simulink model "BEV_system_model"  (R2023a)
settings: Solver=daessc  StartTime=0  StopTime=2474  MaxStep=0.1  RelTol=1e-3  AbsTol=1e-3  EnableMultiTasking=on
PreLoadFcn:
  | defineBus_HighVoltage
  | defineBus_Rotational
PostLoadFcn:
  | BEV_setup
undefined symbols (not defined in the file): Ion, Lithium, Minus, Plus
libraries: spsMosfetLib x4, slpidlib x4, spsCurrentMeasurementLib x2, spsSeriesRLCBranchLib x2, spsVoltageMeasurementLib x2, nesl_utility x2, spsBatteryLib x1, fl_lib x1, simulink x1, spsSupercapacitorLib x1, spspowerguiLib x1
Description:
  | Battery Electric Vehicle drive cycle simulation
settings Model: Creator=MathWorks  LastModifiedBy=antaeug
settings SolverCC: AutoScaleAbsTol=off  AlgebraicLoopSolver=TrustRegion  MinimalZcImpactIntegration=on
settings DataIOCC: MaxDataPoints=15000  SaveFormat=Array  DSMLogging=off
settings OptimizationCC: ReuseModelBlockBuffer=off  ExpressionDepthLimit=2147483647  LifeSpan=inf
settings DebuggingCC: UnderspecifiedInitializationDetection=Classic  MergeDetectMultiDrivingBlocksExec=none  FcnCallInpInsideContextMsg=warning  UnconnectedInputMsg=warning  UnconnectedOutputMsg=warning  UnconnectedLineMsg=warning  StateNameClashWarn=warning  SFUnexpectedBacktrackingDiag=warning  SFNoUnconditionalDefaultTransitionDiag=warning  SFExecutionAtInitializationDiag=none  UnitsInconsistencyMsg=none  ArithmeticOperatorsInVariantConditions=warning
settings HardwareCC: ProdBitPerPointer=32  ProdBitPerSizeT=32  ProdBitPerPtrDiffT=32  ProdLargestAtomicFloat=None  ProdIntDivRoundTo=Undefined  ProdEndianess=Unspecified  ProdWordSize=32  ProdHWDeviceType=32-bit Generic
settings ModelReferenceCC: EnableRefExpFcnMdlSchedulingChecks=on  PropagateSignalLabelsOutOfModel=off
settings SFSimCC: SimUseLocalCustomCode=off  CustomCodeUndefinedFunction=UseInterfaceOnly
settings RTWCC: RTWUseLocalCustomCode=off  DLArmComputeVersion=19.05
settings CodeAppCC: StateflowObjectComments=on
settings GRTTargetCC: TargetLangStandard=C89/C90 (ANSI)  CombineOutputUpdateFcns=off  GRTInterface=on
settings ConfigComp: CovScope=Subsystem  CovPath=Driver & Environment/Torque Limiter  CovMetricSettings=dcmw  CovSaveCumulativeToWorkspaceVar=on  CovSaveSingleToWorkspaceVar=on  CovExternalEMLEnable=off
settings SimscapeCC: SimscapeNominalValues="[{\"value\":\"20\",\"unit\":\"A\"},{\"value\":\"1\",\"unit\":\"bar\"},{\"value\":\"1\",\"unit\":\"cm^2\"},{\"value\":\"1\",\"unit\":\"cm^3/s\"},{\"value\":\"1\",\"unit\":\"kJ/kg\"},{\"value\":\"1\",\"unit\":\"kW\"},{\"value\":\"1\",\"unit\":\"l\"},{\"value\":\"1\",\"unit\":\"N\"},{\"value\":\"40\",\"unit\":\"N*m\"},{\"value\":\"350\",\"unit\":\"V\"}]"  SimscapeLogType=all  SimscapeLogSimulationStatistics=on  SimscapeLogName=logoutssc  SimscapeLogLimitData=off  SimscapeLogDataHistory=10000

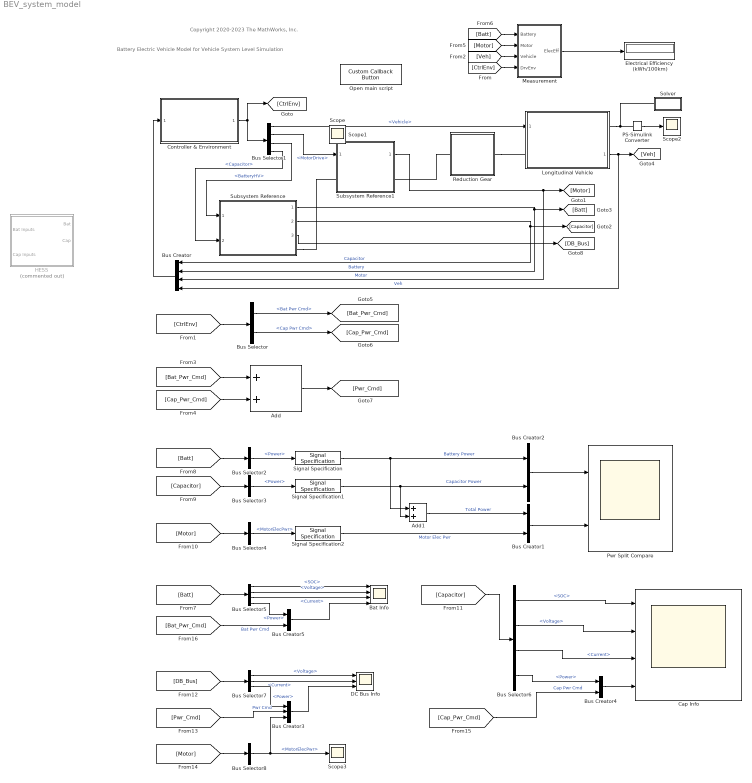
== system BEV_system_model ==
  note: Battery Electric Vehicle Model for Vehicle System Level Simulation
  note: Copyright 2020-2023 The MathWorks, Inc.
  Add : Sum
  Add1 : Sum
  Bat Info : Scope  NumInputPorts=4
  Bus Creator : BusCreator  Inputs=4
  Bus Creator{1..2,4..5} (4 alike) : BusCreator  Inputs=2
  Bus Creator3 : BusCreator  Inputs=3
  Bus Selector : BusSelector  OutputSignals=BatteryHV.Bat Pwr Cmd,Capacitor.Cap Pwr Cmd
  Bus Selector1 : BusSelector  OutputSignals=Vehicle,MotorDrive,BatteryHV,Capacitor
  Bus Selector2 : BusSelector  OutputSignals=Power
  Bus Selector3 : BusSelector  OutputSignals=Power
  Bus Selector4 : BusSelector  OutputSignals=MotorElecPwr
  Bus Selector5 : BusSelector  OutputSignals=SOC,Voltage,Current,Power
  Bus Selector6 : BusSelector  OutputSignals=SOC,Voltage,Current,Power
  Bus Selector7 : BusSelector  OutputSignals=Voltage,Current,Power
  Bus Selector8 : BusSelector  OutputSignals=MotorElecPwr
  Cap Info : Scope  NumInputPorts=4
  Controller & Environment : Subsystem  ReferencedSubsystem=CtrlEnv_refsub_Basic
      settings: OpenFcn=|
      | % Look under mask:
      | open_system(gcb, "force")
  DC Bus Info : Scope  NumInputPorts=3
  Electrical Efficiency (kWh/100km) : Display
  HESS : Subsystem  Commented=on
  Longitudinal Vehicle : Subsystem  ReferencedSubsystem=Vehicle1D_refsub_Basic
      settings: PortSchema="{\"entries\":[{\"content\":{\"sides\":[{\"content\":{\"connectorIds\":[\"In1\",\"LConn1\"]},\"type\":\"ConnectorPlacement.EquallySpacedRectSide\",\"uuid\":\"1278221b-4210-4fc4-9018-d7f4555b8d65\"},{\"content\":{\"connectorIds\":[\"RConn1\",\"Out1\"],\"side\":\"RIGHT\"},\"type\":\"ConnectorPlacement.EquallySpacedRectSide\",\"uuid\":\"ae02a7d1-22cf-4294-9907-02c3616e735c\"},{\"content\":{\"side\":\"TOP\"},\"type\":\"ConnectorPlacement.EquallySpacedRectSide\",\"uuid\":\"498bee53-b001-4331-968a-8dad39da1579\"}]},\"type\":\"ConnectorPlacement.EquallySpacedConnector\",\"uuid\":\"c28a1585-5582-45c2-8974-ffffcb6069ab\"}],\"packageUris\":[\"http://schema.mathworks.com/mf0/Connector/R2020b\"],\"version\":\"1.0\"}"
      settings: OpenFcn=|
      | % Look under mask:
      | open_system(gcb, "force")
  Measurement : Subsystem
  Open main script : CustomCallbackButton  Configuration="{\"components\":[{\"name\":\"BackgroundImageComponent\",\"settings\":{\"image\":{\"size\":[0,0],\"src\":\"default\",\"srcOrientation\":\"Right\"},\"position\":[0,0,1,1]}},{\"name\":\"ButtonStateComponent\",\"settings\":{\"buttonType\":\"momentary\",\"clickFcn\":\"edit(\\\"BEV_main_script\\\")\\n\",\"onValue\":1,\"position\":[0,0,1,1],\"pressDelay\":\"500\",\"pressFcn\":\"\",\"repeatInterval\":\"0\",\"states\":[{\"horizontalAlignment\":\"center\",\"image\":{\"position\":[0,0,1,1],\"src\":\"default\",\"srcOrientation\":\"Right\"},\"label\":{\"color\":[0.01176470588,0.01176470588,0.01176470588,1],\"icon\":{\"size\":[0,0],\"src\":\"default\",\"srcOrientation\":\"Right\"},\"iconPlacement\":\"left\",\"text\":{\"content\":\"Main script\"}},\"labelOffset\":[0,0],\"verticalAlignment\":\"middle\"},{\"horizontalAlignment\":\"center\",\"image\":{\"position\":[0,0,1,1],\"src\":\"default\",\"srcOrientation\":\"Right\"},\"label\":{\"color\":[0.01176470588,0.01176470588,0.01176470588,1],\"icon\":{\"size\":[0,0],\"src\":\"default\",\"srcOrientation\":\"Right\"},\"iconPlacement\":\"left\",\"text\":{\"content\":\"Main script\"}},\"labelOffset\":[0,0],\"verticalAlignment\":\"middle\"},{\"horizontalAlignment\":\"center\",\"image\":{\"position\":[0,0,1,1],\"src\":\"default\",\"srcOrientation\":\"Right\"},\"label\":{\"color\":[0.01176470588,0.01176470588,0.01176470588,1],\"icon\":{\"size\":[0,0],\"src\":\"default\",\"srcOrientation\":\"Right\"},\"iconPlacement\":\"left\",\"text\":{\"content\":\"Main script\"}},\"labelOffset\":[0,0],\"verticalAlignment\":\"middle\"},{\"horizontalAlignment\":\"center\",\"image\":{\"position\":[0,0,1,1],\"src\":\"default\",\"srcOrientation\":\"Right\"},\"label\":{\"color\":[0.01176470588,0.01176470588,0.01176470588,1],\"icon\":{\"size\":[0,0],\"src\":\"default\",\"srcOrientation\":\"Right\"},\"iconPlacement\":\"left\",\"text\":{\"content\":\"Main script\"}},\"labelOffset\":[0,0],\"verticalAlignment\":\"middle\"}]}},{\"name\":\"ForegroundImageComponent\",\"settings\":{\"image\":{\"size\":[0,0],\"src\":\"default\",\"srcOrientation\":\"Right\"},\"isForeground\":1,\"position\":[0,0,1,1]}}],\"settings\":{\"BindingType\":\"standalone\",\"backgroundColor\":[244,244,244,1],\"backgroundOffset\":0.2,\"backgroundOpacity\":1,\"fixedAspectRatio\":\"off\",\"foregroundColor\":[0.01176470588,0.01176470588,0.01176470588,1],\"migratedFromLegacy\":true,\"useBackgroundColor\":true,\"variant\":\"callback\",\"version\":\"R2023a\"},\"type\":\"Button\"}"  CustomBackgroundColor="{\"color\":[0.9568627451,0.9568627451,0.9568627451],\"show\":true}"
  PS-Simulink Converter : nesl_utility/PS-Simulink Converter  PhysicalDomain=network_engine_domain  SubClassName=ps_output  LeftPortType=input  RightPortType=output  PseudoPeriodic=off  Frequencies=[]  VectorFormat=inherit  Unit=m/s  AffineConversion=off
  Pwr Split Compare : Scope  NumInputPorts=2
  Reduction Gear : Subsystem  ReferencedSubsystem=Reducer_refsub_Basic
      settings: OpenFcn=|
      | % Look under mask:
      | open_system(gcb, "force")
  Scope{,1..3} (4 alike) : Scope
  Signal Specification : SignalSpecification  Unit=W
  Signal Specification1 : SignalSpecification  Unit=W
  Signal Specification2 : SignalSpecification  Unit=W
  Solver : Subsystem
  Subsystem Reference : Subsystem  ReferencedSubsystem=BatteryHV_refsub_System
  Subsystem Reference1 : Subsystem  ReferencedSubsystem=MotorDriveUnit_refsub_System
  wires:
  [Veh] -> Measurement/3(Vehicle)
  [Motor] -> Measurement/2(Motor)
  [Batt] -> Measurement/1(Battery)
  Subsystem Reference/1 -> Bus Creator/2, [Batt]  "Battery"
  Longitudinal Vehicle/1 -> [Veh], Bus Creator/4  "Veh"
  [CtrlEnv] -> Measurement/4(DrvEnv)
  Bus Selector1/2 -> Subsystem Reference1/1  "<MotorDrive>"
  Subsystem Reference1/1 -> Bus Creator/3, [Motor]  "Motor"
  Bus Creator/1 -> Controller & Environment/1
  Bus Selector1/3 -> Subsystem Reference/1  "<BatteryHV>"
  Bus Selector1/1 -> Longitudinal Vehicle/1  "<Vehicle>"
  Measurement/1(ElecEff) -> Electrical Efficiency (kWh/100km)/1
  Controller & Environment/1 -> Bus Selector1/1, [CtrlEnv]
  PS-Simulink Converter/1 -> Scope2/1
  Subsystem Reference/2 -> Bus Creator/1, [Capacitor]  "Capacitor"
  Bus Selector1/4 -> Subsystem Reference/2  "<Capacitor>"
  [CtrlEnv] -> Bus Selector/1
  Bus Selector/1 -> [Bat_Pwr_Cmd]  "<Bat Pwr Cmd>"
  Bus Selector/2 -> [Cap_Pwr_Cmd]  "<Cap Pwr Cmd>"
  [Bat_Pwr_Cmd] -> Add/1
  [Cap_Pwr_Cmd] -> Add/2
  Add/1 -> [Pwr_Cmd]
  [Batt] -> Bus Selector2/1
  [Capacitor] -> Bus Selector3/1
  Bus Selector2/1 -> Signal Specification/1  "<Power>"
  Bus Selector3/1 -> Signal Specification1/1  "<Power>"
  Add1/1 -> Bus Creator1/1  "Total Power"
  Bus Creator2/1 -> Pwr Split Compare/1
  Signal Specification/1 -> Add1/1, Bus Creator2/1  "Battery Power"
  Signal Specification1/1 -> Bus Creator2/2, Add1/2  "Capacitor Power"
  Bus Creator1/1 -> Pwr Split Compare/2
  [Motor] -> Bus Selector4/1
  Bus Selector4/1 -> Signal Specification2/1  "<MotorElecPwr>"
  Signal Specification2/1 -> Bus Creator1/2  "Motor Elec Pwr"
  [Batt] -> Bus Selector5/1
  Bus Selector5/2 -> Bat Info/2  "<Voltage>"
  Bus Selector5/1 -> Bat Info/1  "<SOC>"
  Bus Selector5/3 -> Bat Info/3  "<Current>"
  [Capacitor] -> Bus Selector6/1
  Subsystem Reference/3 -> [DB_Bus]
  [DB_Bus] -> Bus Selector7/1
  Bus Selector7/1 -> DC Bus Info/1  "<Voltage>"
  Bus Selector7/2 -> DC Bus Info/2  "<Current>"
  Bus Creator3/1 -> DC Bus Info/3
  Bus Selector7/3 -> Bus Creator3/1  "<Power>"
  [Pwr_Cmd] -> Bus Creator3/2  "Pwr Cmd"
  [Motor] -> Bus Selector8/1
  Bus Selector8/1 -> Bus Creator3/3, Scope3/1  "<MotorElecPwr>"
  Bus Selector6/1 -> Cap Info/1  "<SOC>"
  Bus Selector6/2 -> Cap Info/2  "<Voltage>"
  Bus Selector6/3 -> Cap Info/3  "<Current>"
  Bus Selector6/4 -> Bus Creator4/1  "<Power>"
  [Cap_Pwr_Cmd] -> Bus Creator4/2  "Cap Pwr Cmd"
  Bus Creator4/1 -> Cap Info/4
  Bus Selector5/4 -> Bus Creator5/1  "<Power>"
  Bus Creator5/1 -> Bat Info/4
  [Bat_Pwr_Cmd] -> Bus Creator5/2  "Bat Pwr Cmd"
  connections:
  Reduction Gear/RConn1 -- Longitudinal Vehicle/LConn1
  Reduction Gear/LConn1 -- Subsystem Reference1/RConn1
  Longitudinal Vehicle/RConn1 -- Solver/LConn1 -- PS-Simulink Converter/LConn1
  Subsystem Reference/RConn1 -- Subsystem Reference1/LConn1

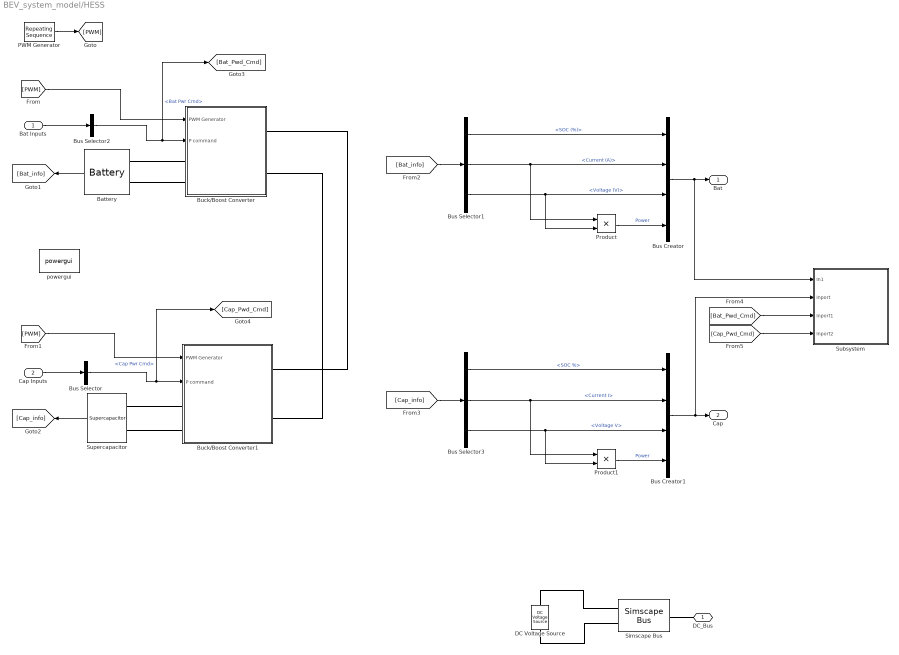
== system BEV_system_model/HESS ==
  Bat Inputs : Inport
  Cap Inputs : Inport  Port=2
  Battery : spsBatteryLib/Battery  BatType=Lithium-Ion  ShowTempParam=off  ThermalPreset=no  ShowAgeParam=off  NomV=300  NomQ=93.6  SOC=100  Batt_Tr=30  PresetModel=on  MaxQ=93.6  MinV=225  FullV=349.1961  Dis_rate=40.6957  R=0.032051  Normal_OP=84.647  expZone="[324.1158      4.598609]"  current=[6.5 13 32.5]  Units=Time  Tci=20  NomT=20  T2=-30  MaxQ2=4.8  FullV2=7.1  Normal_OP2=5.655  expZone2="[6.58           1]"  Rca=0.6  ti=2000  Dp=0  Neq0=0  Tsim=1e6  Ta1=25  Qeol=5.4*0.9  Reol=0.013333*1.2  Char_age=[2.3478, 3]  Dis_age=[2.3478, 10]  N1=1500  N2=10500  N3=1000  N4=1400  Ta2=45  N5=950
  Buck/Boost Converter : Subsystem
  Buck/Boost Converter1 : Subsystem
  Bus Creator : BusCreator  Inputs=4
  Bus Creator1 : BusCreator  Inputs=4
  Bus Selector : BusSelector  OutputSignals=Cap Pwr Cmd
  Bus Selector1 : BusSelector  OutputSignals=SOC (%),Current (A),Voltage (V)
  Bus Selector2 : BusSelector  OutputSignals=Bat Pwr Cmd
  Bus Selector3 : BusSelector  OutputSignals=SOC %,Current I,Voltage V
  DC Voltage Source : fl_lib/Electrical/Electrical Sources/DC Voltage Source  v0=300 V
  PWM Generator : simulink/Sources/Repeating Sequence  rep_seq_t="[0 1/4*0.0001  2/4*0.0001  3/4*0.0001  0.0001]"  rep_seq_y=[0 1 0 -1 0]
  Product : Product
  Product1 : Product
  Simscape Bus : SimscapeBus  HierarchyStrings=Plus;Minus  ConnectionType=Bus: Bus_HighVoltage
  Subsystem : Subsystem
  Supercapacitor : spsSupercapacitorLib/Supercapacitor  C=1500  Rdc=0.00047  Voltage=2.7  Ns=222  Np=1  Vinit=2.7  Temp=25  PresetModel=off  EstParam=off  Nc=1  r=1e-9  epsilon=6.0208e-10  Ich=10  Vstern="[0.161  2.7  7.8]"  Self_dis=on  Ioc=10  Vself="[48  47.8  47.06  44.65]"  demandeplot=off  I="[10  20 100  500]"  Units=sec  Vmax=0  If=0  deltaV=0  alpha=0  sec=0
      settings: LibrarySourceBlock=sps_lib/Sources/Supercapacitor
  powergui : spspowerguiLib/powergui  Priority=1  SimulationMode=Discrete  SampleTime=25e-6  frequency=60  Iterations=50  frequencyindice=0  Pbase=100e6  ErrMax=1e-4  UnitsV=kV  UnitsW=MW  buscounter=0  FunctionMessages=off  echomessages=off  EnableUseOfTLC=off  CurrentSourceSwitches=off  DisableSnubberDevices=off  DisableRonSwitches=off  DisableVfSwitches=off  DisplayEquations=off  AutomaticDiscreteSolvers=off  SolverType=Tustin/Backward Euler (TBE)  Interpol=off  ExternalGateDelay=off  methode=off  Ts=0  x0status=blocks  SPID=off  SwTol=0  HookPort=off  NonlinearTolerance=1e-4  nMaxIteration=100  ContinueOnMaxIteration=off  RestoreLinks=warning  ResistiveCurrentMeasurement=off  Frange=[0:1:1000]  Ylog=on  Xlog=on  ShowGrid=on  save=on  variable=ZDa  structure=donnee  ZoomFFT=off  StartTime=0.0  cycles=1  DisplayStyle=1  fundamental=60  FreqAxis=off  MaxFrequency=1000  frequencyindicesteady=10  RmsSteady=1  display=off
  DC_Bus : PMIOPort  Side=Right
  Bat : Outport
  Cap : Outport  Port=2
  wires:
  Bat Inputs/1 -> Bus Selector2/1
  Cap Inputs/1 -> Bus Selector/1
  PWM Generator/1 -> [PWM]
  Battery/1 -> [Bat_info]
  Supercapacitor/1 -> [Cap_info]
  Bus Selector2/1 -> [Bat_Pwd_Cmd], Buck/Boost Converter/2(P command)  "<Bat Pwr Cmd>"
  [PWM] -> Buck/Boost Converter/1(PWM Generator)
  Bus Selector/1 -> [Cap_Pwd_Cmd], Buck/Boost Converter1/2(P command)  "<Cap Pwr Cmd>"
  [PWM] -> Buck/Boost Converter1/1(PWM Generator)
  [Bat_info] -> Bus Selector1/1
  Bus Creator/1 -> Subsystem/1(In1), Bat/1
  Bus Selector1/1 -> Bus Creator/1  "<SOC (%)>"
  Bus Selector1/2 -> Product/1, Bus Creator/2  "<Current (A)>"
  Bus Selector1/3 -> Product/2, Bus Creator/3  "<Voltage (V)>"
  [Cap_info] -> Bus Selector3/1
  Bus Selector3/3 -> Product1/2, Bus Creator1/3  "<Voltage V>"
  Bus Selector3/2 -> Product1/1, Bus Creator1/2  "<Current I>"
  Product1/1 -> Bus Creator1/4  "Power"
  Bus Selector3/1 -> Bus Creator1/1  "<SOC %>"
  Bus Creator1/1 -> Subsystem/2(Inport), Cap/1
  [Bat_Pwd_Cmd] -> Subsystem/3(Inport1)
  [Cap_Pwd_Cmd] -> Subsystem/4(Inport2)
  Product/1 -> Bus Creator/4  "Power"
  connections:
  DC_Bus/RConn1 -- Simscape Bus/RConn1
  Buck/Boost Converter/LConn1 -- Battery/LConn1
  Buck/Boost Converter/LConn2 -- Battery/LConn2
  Buck/Boost Converter1/LConn1 -- Supercapacitor/LConn1
  Supercapacitor/LConn2 -- Buck/Boost Converter1/LConn2
  Buck/Boost Converter/RConn1 -- Buck/Boost Converter1/RConn1
  Buck/Boost Converter/RConn2 -- Buck/Boost Converter1/RConn2
  DC Voltage Source/LConn1 -- Simscape Bus/LConn1
  DC Voltage Source/RConn1 -- Simscape Bus/LConn2

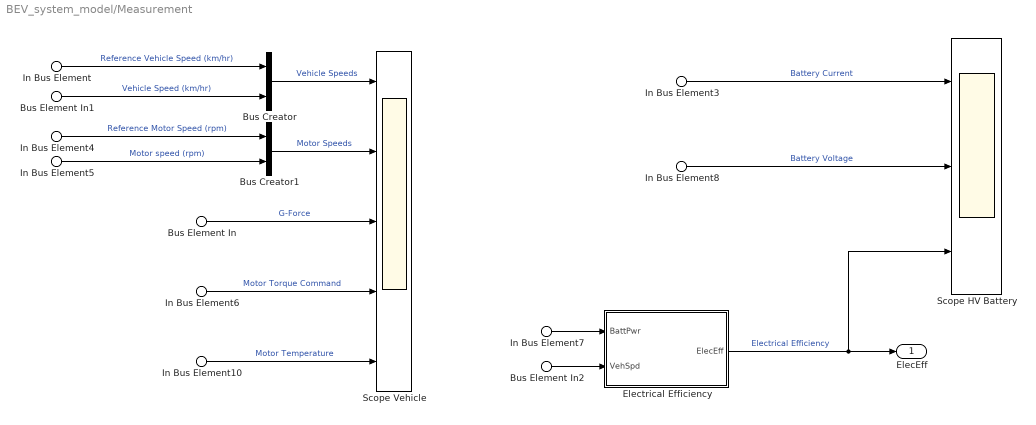
== system BEV_system_model/Measurement ==
  In Bus Element3 : Inport  PortName=Battery  Element=Current
  In Bus Element7 : Inport  PortName=Battery  Element=Power
  In Bus Element8 : Inport  PortName=Battery  Element=Voltage
  In Bus Element6 : Inport  Port=2  PortName=Motor  Element=TrqCmd
  In Bus Element5 : Inport  Port=2  PortName=Motor  Element=MotorSpd
  In Bus Element10 : Inport  Port=2  PortName=Motor  Element=MotorTemp
  Bus Element In : Inport  Port=3  PortName=Vehicle  Element=G
  Bus Element In2 : Inport  Port=3  PortName=Vehicle  Element=VehSpdKph
  Bus Element In1 : Inport  Port=3  PortName=Vehicle  Element=VehSpdKph
  In Bus Element : Inport  Port=4  PortName=DrvEnv  Element=Info.VehSpdRef
  In Bus Element4 : Inport  Port=4  PortName=DrvEnv  Element=Info.MotorSpdRef
  Bus Creator : BusCreator  Inputs=2
  Bus Creator1 : BusCreator  Inputs=2
  Electrical Efficiency : Subsystem
  Scope HV Battery : Scope  NumInputPorts=3
  Scope Vehicle : Scope  NumInputPorts=5
  ElecEff : Outport
  wires:
  In Bus Element3/1 -> Scope HV Battery/1  "Battery Current"
  In Bus Element/1 -> Bus Creator/1  "Reference Vehicle Speed (km/hr)"
  Bus Element In1/1 -> Bus Creator/2  "Vehicle Speed (km/hr)"
  In Bus Element5/1 -> Bus Creator1/2  "Motor speed (rpm)"
  In Bus Element4/1 -> Bus Creator1/1  "Reference Motor Speed (rpm)"
  Bus Creator1/1 -> Scope Vehicle/2  "Motor Speeds"
  Bus Element In/1 -> Scope Vehicle/3  "G-Force"
  Bus Creator/1 -> Scope Vehicle/1  "Vehicle Speeds"
  In Bus Element6/1 -> Scope Vehicle/4  "Motor Torque Command"
  In Bus Element10/1 -> Scope Vehicle/5  "Motor Temperature"
  In Bus Element8/1 -> Scope HV Battery/2  "Battery Voltage"
  Electrical Efficiency/1(ElecEff) -> Scope HV Battery/3, ElecEff/1  "Electrical Efficiency"
  In Bus Element7/1 -> Electrical Efficiency/1(BattPwr)
  Bus Element In2/1 -> Electrical Efficiency/2(VehSpd)

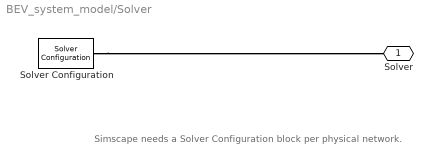
== system BEV_system_model/Solver ==
  note: Simscape needs a Solver Configuration block per physical network.
  Solver Configuration : nesl_utility/Solver Configuration  PhysicalDomain=network_engine_domain  SubClassName=solver  LeftPortType=input  RightPortType=generic  Tones=[]  Harmonics=[]  SimulateNoise=off  Profile=off  UseLocalSampling=off  EnableSwitchedLinearOptims=on  FrequencyDomain=off  UseCCode=off  RelTol=0.001  AbsTol=1e-06  MinStep=1e-09  ToWorkspace=off  RevertToSquareIcSolve=off  NumHomotopyIterations=100  PhasorMode=off  PhasorModeNumHarmonics=1  ConsistencySolver=NEWTON_FTOL  IndexReductionMethod=DerivativeReplacement  DoDC=off  ResidualTolerance=1e-6  ConsistencyTolSource=GLOBAL  ConsistencyAbsTol=0.001  ConsistencyRelTol=0.001  ConsistencyTolFactor=0.001  UseLocalSolver=off  LocalSolverChoice=NE_BACKWARD_EULER_ADVANCER  ResolveIndetEquations=on  FunctionEvalNumThread=1  LocalSolverSampleTime=0.01  DoFixedCost=off  MaxNonlinIter=3  MaxModeIter=2  ComputeImpulses=off  ImpulseIterations=2  LinearAlgebra=auto  LinearAlgebraNumThread=0  EquationFormulation=NE_TIME_EF  DelaysMemoryBudget=1024  AutomaticFiltering=on  FilteringTimeConstant=0.001  PartitionStorageMethod=AS_NEEDED  PartitionMemoryBudget=1024  PartitionMethod=FAST
      settings: AttributesFormatString=Local solver %<UseLocalSolver>
  Solver : PMIOPort  Side=Left
  connections:
  Solver Configuration/RConn1 -- Solver/RConn1

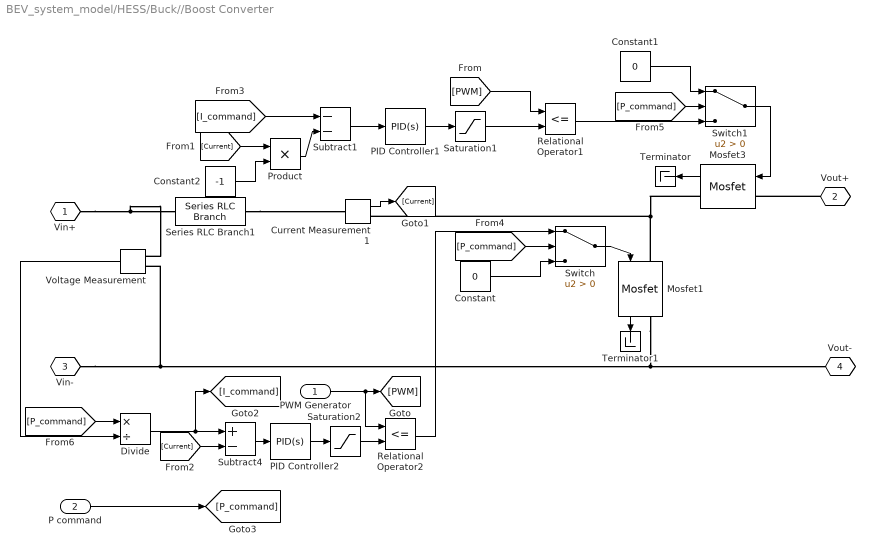
== system BEV_system_model/HESS/Buck//Boost Converter ==
  PWM Generator : Inport
  P command : Inport  Port=2
  Constant : Constant  Value=0
  Constant1 : Constant  Value=0
  Constant2 : Constant  Value=-1
  Current Measurement1 : spsCurrentMeasurementLib/Current Measurement  PhasorSimulation=off  OutputType=Complex  PSBequivalent=0
  Divide : Product  Inputs=*/
  Mosfet1 : spsMosfetLib/Mosfet  Ron=0.1  Lon=0  Rd=0.01  Vfd=0  IC=0  Rs=1e5  Cs=inf  Measurements=on
  Mosfet3 : spsMosfetLib/Mosfet  Ron=0.1  Lon=0  Rd=0.01  Vfd=0  IC=0  Rs=1e5  Cs=inf  Measurements=on
  PID Controller1 : slpidlib/PID Controller  Controller=PID  Form=Parallel  TimeDomain=Continuous-time  UseExternalTs=off  SampleTime=-1  IntegratorMethod=Forward Euler  FilterMethod=Forward Euler  ControllerParametersSource=internal  P=1.5  I=1  UseKiTs=off  D=0  N=100  UseFilter=on  TunerSelectOption=Transfer Function Based (PID Tuner App)  InitialConditionSource=internal  InitialConditionForIntegrator=0  InitialConditionForFilter=0  DifferentiatorICPrevScaledInput=0  ExternalReset=none  TrackingMode=off  Kt=1  LimitOutput=off  SatLimitsSource=internal  UpperSaturationLimit=inf  LowerSaturationLimit=-inf  LinearizeAsGain=off  AntiWindupMode=none  Kb=1  LimitIntegrator=off  UpperIntegratorSaturationLimit=inf  LowerIntegratorSaturationLimit=-inf  POutMin=[]  POutMax=[]  IOutMin=[]  IOutMax=[]  DOutMin=[]  DOutMax=[]  NOutMin=[]  NOutMax=[]  SumOutMin=[]  SumOutMax=[]  SaturationOutMin=[]  SaturationOutMax=[]  PParamMin=[]  PParamMax=[]  IParamMin=[]  IParamMax=[]  DParamMin=[]  DParamMax=[]  NParamMin=[]  NParamMax=[]  KbParamMin=[]  KbParamMax=[]  KtParamMin=[]  KtParamMax=[]  KbOutMin=[]  KbOutMax=[]  KtOutMin=[]  KtOutMax=[]  IntegratorOutMin=[]  IntegratorOutMax=[]  FilterOutMin=[]  FilterOutMax=[]  SumI1OutMin=[]  SumI1OutMax=[]  SumI2OutMin=[]  SumI2OutMax=[]  SumI3OutMin=[]  SumI3OutMax=[]  SumI4OutMin=[]  SumI4OutMax=[]  SumDOutMin=[]  SumDOutMax=[]  DifferentiatorOutMin=[]  DifferentiatorOutMax=[]  FilterDiffOutCoefMin=[]  FilterDiffOutCoefMax=[]  ReciprocalOutMin=[]  ReciprocalOutMax=[]  SumDenOutMin=[]  SumDenOutMax=[]  SumNumOutMin=[]  SumNumOutMax=[]  DivideOutMin=[]  DivideOutMax=[]  UdiffTsProdOutMin=[]  UdiffTsProdOutMax=[]  NTsProdOutMin=[]  NTsProdOutMax=[]  UintegralTsProdOutMin=[]  UintegralTsProdOutMax=[]  UngainTsProdOutMin=[]  UngainTsProdOutMax=[]  ClampingZeroOutDataTypeStr=Inherit: Inherit via back propagation  ClampingZeroOutMin=[]  ClampingZeroOutMax=[]  FilterDenConstantOutDataTypeStr=Inherit: Inherit via back propagation  FilterDenConstantOutMin=[]  FilterDenConstantOutMax=[]  PCopyOutDataTypeStr=Inherit: Inherit via back propagation  PCopyOutMin=[]  PCopyOutMax=[]  NCopyOutDataTypeStr=Inherit: Inherit via back propagation  NCopyOutMin=[]  NCopyOutMax=[]  IntegratorContinuousStateAttributes=''  IntegratorStateMustResolveToSignalObject=off  IntegratorRTWStateStorageClass=Auto  FilterContinuousStateAttributes=''  FilterStateMustResolveToSignalObject=off  FilterRTWStateStorageClass=Auto  ParallelPVariant=InternalParameters  IdealPVariant=Disabled  IVariant=InternalParameters  DVariant=InternalParameters  IntegratorVariant=Continuous  SatVariant=Disabled  AWVariant=Passthrough  PCopyVariant=Disabled  TRVariant=Disabled  FdbkBlocksVariant=Forward  IdealPFdbkVariant=Disabled  SatFdbkVariant=Disabled  DerivativeFilterVariant=ContFilter  NVariant=InternalParameters  NCopyVariant=Disabled  FilterICVariant=InternalICsFilter  IntegratorICVariant=InternalICs  ExternalResetVariant=Disabled  TRSumVariant=Passthrough  SumFdbkVariant=Disabled  SumVariant=Sum_PID  TsampFilterVariant=InternalTs  TsampNgainVariant=Passthrough  TsampIntegralVariant=Disabled_SignalSpec  ExternalSaturationOutDataTypeStr=Inherit: Same as second input
  PID Controller2 : slpidlib/PID Controller  Controller=PID  Form=Parallel  TimeDomain=Continuous-time  UseExternalTs=off  SampleTime=-1  IntegratorMethod=Forward Euler  FilterMethod=Forward Euler  ControllerParametersSource=internal  P=1.5  I=1  UseKiTs=off  D=0  N=100  UseFilter=on  TunerSelectOption=Transfer Function Based (PID Tuner App)  InitialConditionSource=internal  InitialConditionForIntegrator=0  InitialConditionForFilter=0  DifferentiatorICPrevScaledInput=0  ExternalReset=none  TrackingMode=off  Kt=1  LimitOutput=off  SatLimitsSource=internal  UpperSaturationLimit=inf  LowerSaturationLimit=-inf  LinearizeAsGain=off  AntiWindupMode=none  Kb=1  LimitIntegrator=off  UpperIntegratorSaturationLimit=inf  LowerIntegratorSaturationLimit=-inf  POutMin=[]  POutMax=[]  IOutMin=[]  IOutMax=[]  DOutMin=[]  DOutMax=[]  NOutMin=[]  NOutMax=[]  SumOutMin=[]  SumOutMax=[]  SaturationOutMin=[]  SaturationOutMax=[]  PParamMin=[]  PParamMax=[]  IParamMin=[]  IParamMax=[]  DParamMin=[]  DParamMax=[]  NParamMin=[]  NParamMax=[]  KbParamMin=[]  KbParamMax=[]  KtParamMin=[]  KtParamMax=[]  KbOutMin=[]  KbOutMax=[]  KtOutMin=[]  KtOutMax=[]  IntegratorOutMin=[]  IntegratorOutMax=[]  FilterOutMin=[]  FilterOutMax=[]  SumI1OutMin=[]  SumI1OutMax=[]  SumI2OutMin=[]  SumI2OutMax=[]  SumI3OutMin=[]  SumI3OutMax=[]  SumI4OutMin=[]  SumI4OutMax=[]  SumDOutMin=[]  SumDOutMax=[]  DifferentiatorOutMin=[]  DifferentiatorOutMax=[]  FilterDiffOutCoefMin=[]  FilterDiffOutCoefMax=[]  ReciprocalOutMin=[]  ReciprocalOutMax=[]  SumDenOutMin=[]  SumDenOutMax=[]  SumNumOutMin=[]  SumNumOutMax=[]  DivideOutMin=[]  DivideOutMax=[]  UdiffTsProdOutMin=[]  UdiffTsProdOutMax=[]  NTsProdOutMin=[]  NTsProdOutMax=[]  UintegralTsProdOutMin=[]  UintegralTsProdOutMax=[]  UngainTsProdOutMin=[]  UngainTsProdOutMax=[]  ClampingZeroOutDataTypeStr=Inherit: Inherit via back propagation  ClampingZeroOutMin=[]  ClampingZeroOutMax=[]  FilterDenConstantOutDataTypeStr=Inherit: Inherit via back propagation  FilterDenConstantOutMin=[]  FilterDenConstantOutMax=[]  PCopyOutDataTypeStr=Inherit: Inherit via back propagation  PCopyOutMin=[]  PCopyOutMax=[]  NCopyOutDataTypeStr=Inherit: Inherit via back propagation  NCopyOutMin=[]  NCopyOutMax=[]  IntegratorContinuousStateAttributes=''  IntegratorStateMustResolveToSignalObject=off  IntegratorRTWStateStorageClass=Auto  FilterContinuousStateAttributes=''  FilterStateMustResolveToSignalObject=off  FilterRTWStateStorageClass=Auto  ParallelPVariant=InternalParameters  IdealPVariant=Disabled  IVariant=InternalParameters  DVariant=InternalParameters  IntegratorVariant=Continuous  SatVariant=Disabled  AWVariant=Passthrough  PCopyVariant=Disabled  TRVariant=Disabled  FdbkBlocksVariant=Forward  IdealPFdbkVariant=Disabled  SatFdbkVariant=Disabled  DerivativeFilterVariant=ContFilter  NVariant=InternalParameters  NCopyVariant=Disabled  FilterICVariant=InternalICsFilter  IntegratorICVariant=InternalICs  ExternalResetVariant=Disabled  TRSumVariant=Passthrough  SumFdbkVariant=Disabled  SumVariant=Sum_PID  TsampFilterVariant=InternalTs  TsampNgainVariant=Passthrough  TsampIntegralVariant=Disabled_SignalSpec  ExternalSaturationOutDataTypeStr=Inherit: Same as second input
  Product : Product  RndMeth=Zero
  Relational Operator1 : RelationalOperator  Operator=<=  OutDataTypeStr=boolean  InputSameDT=off
  Relational Operator2 : RelationalOperator  Operator=<=  OutDataTypeStr=boolean  InputSameDT=off
  Saturation1 : Saturate  UpperLimit=1  LowerLimit=-1
  Saturation2 : Saturate  UpperLimit=1  LowerLimit=-1
  Series RLC Branch1 : spsSeriesRLCBranchLib/Series RLC Branch  LConnTagsString=__new0  RConnTagsString=__new0  BranchType=L  Resistance=1  Inductance=1e-3  SetiL0=off  InitialCurrent=0  Capacitance=1e-6  Setx0=off  InitialVoltage=0  Measurements=None
  Subtract1 : Sum  Inputs=--
  Subtract4 : Sum  Inputs=+-
  Switch : Switch  Criteria=u2 > Threshold  SaturateOnIntegerOverflow=off  InputSameDT=off
  Switch1 : Switch  Criteria=u2 > Threshold  SaturateOnIntegerOverflow=off  InputSameDT=off
  Terminator : Terminator
  Terminator1 : Terminator
  Voltage Measurement : spsVoltageMeasurementLib/Voltage Measurement  PhasorSimulation=off  OutputType=Complex  PSBequivalent=0
  Vin+ : PMIOPort  Tag=PMCPort  Side=Left
  Vout+ : PMIOPort  Tag=PMCPort  Port=2  Side=Right
  Vin- : PMIOPort  Tag=PMCPort  Port=3  Side=Left
  Vout- : PMIOPort  Tag=PMCPort  Port=4  Side=Right
  wires:
  Saturation2/1 -> Relational Operator2/2
  PID Controller2/1 -> Saturation2/1
  Subtract4/1 -> PID Controller2/1
  PWM Generator/1 -> Relational Operator2/1, [PWM]
  Divide/1 -> [I_command], Subtract4/1
  P command/1 -> [P_command]
  Switch/1 -> Mosfet1/1
  Saturation1/1 -> Relational Operator1/2
  PID Controller1/1 -> Saturation1/1
  Subtract1/1 -> PID Controller1/1
  [PWM] -> Relational Operator1/1
  [Current] -> Subtract4/2
  [Current] -> Product/1
  Product/1 -> Subtract1/2
  Constant2/1 -> Product/2
  [I_command] -> Subtract1/1
  Current Measurement1/1 -> [Current]
  Switch1/1 -> Mosfet3/1
  Relational Operator2/1 -> Switch/1
  Constant/1 -> Switch/3
  Constant1/1 -> Switch1/1
  Mosfet3/1 -> Terminator/1
  Mosfet1/1 -> Terminator1/1
  Relational Operator1/1 -> Switch1/3
  [P_command] -> Switch/2
  [P_command] -> Switch1/2
  [P_command] -> Divide/1
  Voltage Measurement/1 -> Divide/2
  connections:
  Vin-/RConn1 -- Voltage Measurement/LConn2 -- Vout-/RConn1 -- Mosfet1/RConn1
  Vin+/RConn1 -- Series RLC Branch1/LConn1 -- Voltage Measurement/LConn1
  Mosfet1/LConn1 -- Current Measurement1/RConn1 -- Mosfet3/RConn1
  Series RLC Branch1/RConn1 -- Current Measurement1/LConn1
  Vout+/RConn1 -- Mosfet3/LConn1

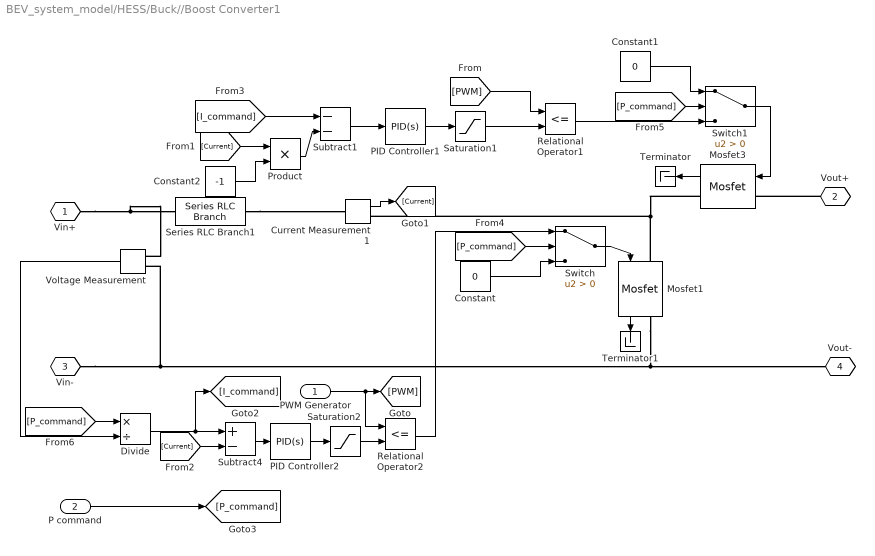
== system BEV_system_model/HESS/Buck//Boost Converter1 ==
  PWM Generator : Inport
  P command : Inport  Port=2
  Constant : Constant  Value=0
  Constant1 : Constant  Value=0
  Constant2 : Constant  Value=-1
  Current Measurement1 : spsCurrentMeasurementLib/Current Measurement  PhasorSimulation=off  OutputType=Complex  PSBequivalent=0
  Divide : Product  Inputs=*/
  Mosfet1 : spsMosfetLib/Mosfet  Ron=0.1  Lon=0  Rd=0.01  Vfd=0  IC=0  Rs=1e5  Cs=inf  Measurements=on
  Mosfet3 : spsMosfetLib/Mosfet  Ron=0.1  Lon=0  Rd=0.01  Vfd=0  IC=0  Rs=1e5  Cs=inf  Measurements=on
  PID Controller1 : slpidlib/PID Controller  Controller=PID  Form=Parallel  TimeDomain=Continuous-time  UseExternalTs=off  SampleTime=-1  IntegratorMethod=Forward Euler  FilterMethod=Forward Euler  ControllerParametersSource=internal  P=1.5  I=1  UseKiTs=off  D=0  N=100  UseFilter=on  TunerSelectOption=Transfer Function Based (PID Tuner App)  InitialConditionSource=internal  InitialConditionForIntegrator=0  InitialConditionForFilter=0  DifferentiatorICPrevScaledInput=0  ExternalReset=none  TrackingMode=off  Kt=1  LimitOutput=off  SatLimitsSource=internal  UpperSaturationLimit=inf  LowerSaturationLimit=-inf  LinearizeAsGain=off  AntiWindupMode=none  Kb=1  LimitIntegrator=off  UpperIntegratorSaturationLimit=inf  LowerIntegratorSaturationLimit=-inf  POutMin=[]  POutMax=[]  IOutMin=[]  IOutMax=[]  DOutMin=[]  DOutMax=[]  NOutMin=[]  NOutMax=[]  SumOutMin=[]  SumOutMax=[]  SaturationOutMin=[]  SaturationOutMax=[]  PParamMin=[]  PParamMax=[]  IParamMin=[]  IParamMax=[]  DParamMin=[]  DParamMax=[]  NParamMin=[]  NParamMax=[]  KbParamMin=[]  KbParamMax=[]  KtParamMin=[]  KtParamMax=[]  KbOutMin=[]  KbOutMax=[]  KtOutMin=[]  KtOutMax=[]  IntegratorOutMin=[]  IntegratorOutMax=[]  FilterOutMin=[]  FilterOutMax=[]  SumI1OutMin=[]  SumI1OutMax=[]  SumI2OutMin=[]  SumI2OutMax=[]  SumI3OutMin=[]  SumI3OutMax=[]  SumI4OutMin=[]  SumI4OutMax=[]  SumDOutMin=[]  SumDOutMax=[]  DifferentiatorOutMin=[]  DifferentiatorOutMax=[]  FilterDiffOutCoefMin=[]  FilterDiffOutCoefMax=[]  ReciprocalOutMin=[]  ReciprocalOutMax=[]  SumDenOutMin=[]  SumDenOutMax=[]  SumNumOutMin=[]  SumNumOutMax=[]  DivideOutMin=[]  DivideOutMax=[]  UdiffTsProdOutMin=[]  UdiffTsProdOutMax=[]  NTsProdOutMin=[]  NTsProdOutMax=[]  UintegralTsProdOutMin=[]  UintegralTsProdOutMax=[]  UngainTsProdOutMin=[]  UngainTsProdOutMax=[]  ClampingZeroOutDataTypeStr=Inherit: Inherit via back propagation  ClampingZeroOutMin=[]  ClampingZeroOutMax=[]  FilterDenConstantOutDataTypeStr=Inherit: Inherit via back propagation  FilterDenConstantOutMin=[]  FilterDenConstantOutMax=[]  PCopyOutDataTypeStr=Inherit: Inherit via back propagation  PCopyOutMin=[]  PCopyOutMax=[]  NCopyOutDataTypeStr=Inherit: Inherit via back propagation  NCopyOutMin=[]  NCopyOutMax=[]  IntegratorContinuousStateAttributes=''  IntegratorStateMustResolveToSignalObject=off  IntegratorRTWStateStorageClass=Auto  FilterContinuousStateAttributes=''  FilterStateMustResolveToSignalObject=off  FilterRTWStateStorageClass=Auto  ParallelPVariant=InternalParameters  IdealPVariant=Disabled  IVariant=InternalParameters  DVariant=InternalParameters  IntegratorVariant=Continuous  SatVariant=Disabled  AWVariant=Passthrough  PCopyVariant=Disabled  TRVariant=Disabled  FdbkBlocksVariant=Forward  IdealPFdbkVariant=Disabled  SatFdbkVariant=Disabled  DerivativeFilterVariant=ContFilter  NVariant=InternalParameters  NCopyVariant=Disabled  FilterICVariant=InternalICsFilter  IntegratorICVariant=InternalICs  ExternalResetVariant=Disabled  TRSumVariant=Passthrough  SumFdbkVariant=Disabled  SumVariant=Sum_PID  TsampFilterVariant=InternalTs  TsampNgainVariant=Passthrough  TsampIntegralVariant=Disabled_SignalSpec  ExternalSaturationOutDataTypeStr=Inherit: Same as second input
  PID Controller2 : slpidlib/PID Controller  Controller=PID  Form=Parallel  TimeDomain=Continuous-time  UseExternalTs=off  SampleTime=-1  IntegratorMethod=Forward Euler  FilterMethod=Forward Euler  ControllerParametersSource=internal  P=1.5  I=1  UseKiTs=off  D=0  N=100  UseFilter=on  TunerSelectOption=Transfer Function Based (PID Tuner App)  InitialConditionSource=internal  InitialConditionForIntegrator=0  InitialConditionForFilter=0  DifferentiatorICPrevScaledInput=0  ExternalReset=none  TrackingMode=off  Kt=1  LimitOutput=off  SatLimitsSource=internal  UpperSaturationLimit=inf  LowerSaturationLimit=-inf  LinearizeAsGain=off  AntiWindupMode=none  Kb=1  LimitIntegrator=off  UpperIntegratorSaturationLimit=inf  LowerIntegratorSaturationLimit=-inf  POutMin=[]  POutMax=[]  IOutMin=[]  IOutMax=[]  DOutMin=[]  DOutMax=[]  NOutMin=[]  NOutMax=[]  SumOutMin=[]  SumOutMax=[]  SaturationOutMin=[]  SaturationOutMax=[]  PParamMin=[]  PParamMax=[]  IParamMin=[]  IParamMax=[]  DParamMin=[]  DParamMax=[]  NParamMin=[]  NParamMax=[]  KbParamMin=[]  KbParamMax=[]  KtParamMin=[]  KtParamMax=[]  KbOutMin=[]  KbOutMax=[]  KtOutMin=[]  KtOutMax=[]  IntegratorOutMin=[]  IntegratorOutMax=[]  FilterOutMin=[]  FilterOutMax=[]  SumI1OutMin=[]  SumI1OutMax=[]  SumI2OutMin=[]  SumI2OutMax=[]  SumI3OutMin=[]  SumI3OutMax=[]  SumI4OutMin=[]  SumI4OutMax=[]  SumDOutMin=[]  SumDOutMax=[]  DifferentiatorOutMin=[]  DifferentiatorOutMax=[]  FilterDiffOutCoefMin=[]  FilterDiffOutCoefMax=[]  ReciprocalOutMin=[]  ReciprocalOutMax=[]  SumDenOutMin=[]  SumDenOutMax=[]  SumNumOutMin=[]  SumNumOutMax=[]  DivideOutMin=[]  DivideOutMax=[]  UdiffTsProdOutMin=[]  UdiffTsProdOutMax=[]  NTsProdOutMin=[]  NTsProdOutMax=[]  UintegralTsProdOutMin=[]  UintegralTsProdOutMax=[]  UngainTsProdOutMin=[]  UngainTsProdOutMax=[]  ClampingZeroOutDataTypeStr=Inherit: Inherit via back propagation  ClampingZeroOutMin=[]  ClampingZeroOutMax=[]  FilterDenConstantOutDataTypeStr=Inherit: Inherit via back propagation  FilterDenConstantOutMin=[]  FilterDenConstantOutMax=[]  PCopyOutDataTypeStr=Inherit: Inherit via back propagation  PCopyOutMin=[]  PCopyOutMax=[]  NCopyOutDataTypeStr=Inherit: Inherit via back propagation  NCopyOutMin=[]  NCopyOutMax=[]  IntegratorContinuousStateAttributes=''  IntegratorStateMustResolveToSignalObject=off  IntegratorRTWStateStorageClass=Auto  FilterContinuousStateAttributes=''  FilterStateMustResolveToSignalObject=off  FilterRTWStateStorageClass=Auto  ParallelPVariant=InternalParameters  IdealPVariant=Disabled  IVariant=InternalParameters  DVariant=InternalParameters  IntegratorVariant=Continuous  SatVariant=Disabled  AWVariant=Passthrough  PCopyVariant=Disabled  TRVariant=Disabled  FdbkBlocksVariant=Forward  IdealPFdbkVariant=Disabled  SatFdbkVariant=Disabled  DerivativeFilterVariant=ContFilter  NVariant=InternalParameters  NCopyVariant=Disabled  FilterICVariant=InternalICsFilter  IntegratorICVariant=InternalICs  ExternalResetVariant=Disabled  TRSumVariant=Passthrough  SumFdbkVariant=Disabled  SumVariant=Sum_PID  TsampFilterVariant=InternalTs  TsampNgainVariant=Passthrough  TsampIntegralVariant=Disabled_SignalSpec  ExternalSaturationOutDataTypeStr=Inherit: Same as second input
  Product : Product  RndMeth=Zero
  Relational Operator1 : RelationalOperator  Operator=<=  OutDataTypeStr=boolean  InputSameDT=off
  Relational Operator2 : RelationalOperator  Operator=<=  OutDataTypeStr=boolean  InputSameDT=off
  Saturation1 : Saturate  UpperLimit=1  LowerLimit=-1
  Saturation2 : Saturate  UpperLimit=1  LowerLimit=-1
  Series RLC Branch1 : spsSeriesRLCBranchLib/Series RLC Branch  LConnTagsString=__new0  RConnTagsString=__new0  BranchType=L  Resistance=1  Inductance=1e-3  SetiL0=off  InitialCurrent=0  Capacitance=1e-6  Setx0=off  InitialVoltage=0  Measurements=None
  Subtract1 : Sum  Inputs=--
  Subtract4 : Sum  Inputs=+-
  Switch : Switch  Criteria=u2 > Threshold  SaturateOnIntegerOverflow=off  InputSameDT=off
  Switch1 : Switch  Criteria=u2 > Threshold  SaturateOnIntegerOverflow=off  InputSameDT=off
  Terminator : Terminator
  Terminator1 : Terminator
  Voltage Measurement : spsVoltageMeasurementLib/Voltage Measurement  PhasorSimulation=off  OutputType=Complex  PSBequivalent=0
  Vin+ : PMIOPort  Tag=PMCPort  Side=Left
  Vout+ : PMIOPort  Tag=PMCPort  Port=2  Side=Right
  Vin- : PMIOPort  Tag=PMCPort  Port=3  Side=Left
  Vout- : PMIOPort  Tag=PMCPort  Port=4  Side=Right
  wires:
  Saturation2/1 -> Relational Operator2/2
  PID Controller2/1 -> Saturation2/1
  Subtract4/1 -> PID Controller2/1
  PWM Generator/1 -> Relational Operator2/1, [PWM]
  Divide/1 -> [I_command], Subtract4/1
  P command/1 -> [P_command]
  Switch/1 -> Mosfet1/1
  Saturation1/1 -> Relational Operator1/2
  PID Controller1/1 -> Saturation1/1
  Subtract1/1 -> PID Controller1/1
  [PWM] -> Relational Operator1/1
  [Current] -> Subtract4/2
  [Current] -> Product/1
  Product/1 -> Subtract1/2
  Constant2/1 -> Product/2
  [I_command] -> Subtract1/1
  Current Measurement1/1 -> [Current]
  Switch1/1 -> Mosfet3/1
  Relational Operator2/1 -> Switch/1
  Constant/1 -> Switch/3
  Constant1/1 -> Switch1/1
  Mosfet3/1 -> Terminator/1
  Mosfet1/1 -> Terminator1/1
  Relational Operator1/1 -> Switch1/3
  [P_command] -> Switch/2
  [P_command] -> Switch1/2
  [P_command] -> Divide/1
  Voltage Measurement/1 -> Divide/2
  connections:
  Vin-/RConn1 -- Voltage Measurement/LConn2 -- Vout-/RConn1 -- Mosfet1/RConn1
  Vin+/RConn1 -- Series RLC Branch1/LConn1 -- Voltage Measurement/LConn1
  Mosfet1/LConn1 -- Current Measurement1/RConn1 -- Mosfet3/RConn1
  Series RLC Branch1/RConn1 -- Current Measurement1/LConn1
  Vout+/RConn1 -- Mosfet3/LConn1

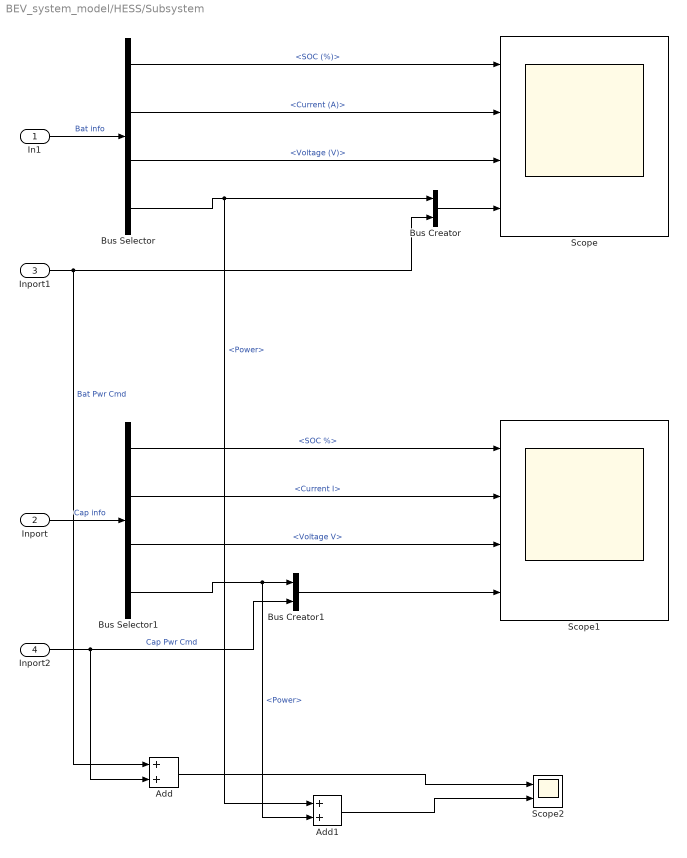
== system BEV_system_model/HESS/Subsystem ==
  In1 : Inport
  Inport : Inport  Port=2
  Inport1 : Inport  Port=3
  Inport2 : Inport  Port=4
  Add : Sum
  Add1 : Sum
  Bus Creator : BusCreator  Inputs=2
  Bus Creator1 : BusCreator  Inputs=2
  Bus Selector : BusSelector  OutputSignals=SOC (%),Current (A),Voltage (V),Power
  Bus Selector1 : BusSelector  OutputSignals=SOC %,Current I,Voltage V,Power
  Scope : Scope  NumInputPorts=4
  Scope1 : Scope  NumInputPorts=4
  Scope2 : Scope  NumInputPorts=2
  wires:
  In1/1 -> Bus Selector/1  "Bat info"
  Inport/1 -> Bus Selector1/1  "Cap info"
  Inport2/1 -> Add/2, Bus Creator1/2  "Cap Pwr Cmd"
  Bus Selector/2 -> Scope/2  "<Current (A)>"
  Bus Selector/1 -> Scope/1  "<SOC (%)>"
  Bus Selector/3 -> Scope/3  "<Voltage (V)>"
  Bus Creator/1 -> Scope/4
  Bus Selector/4 -> Add1/1, Bus Creator/1  "<Power>"
  Bus Selector1/1 -> Scope1/1  "<SOC %>"
  Bus Selector1/2 -> Scope1/2  "<Current I>"
  Bus Selector1/3 -> Scope1/3  "<Voltage V>"
  Bus Creator1/1 -> Scope1/4
  Bus Selector1/4 -> Add1/2, Bus Creator1/1  "<Power>"
  Inport1/1 -> Bus Creator/2, Add/1  "Bat Pwr Cmd"
  Add/1 -> Scope2/1
  Add1/1 -> Scope2/2

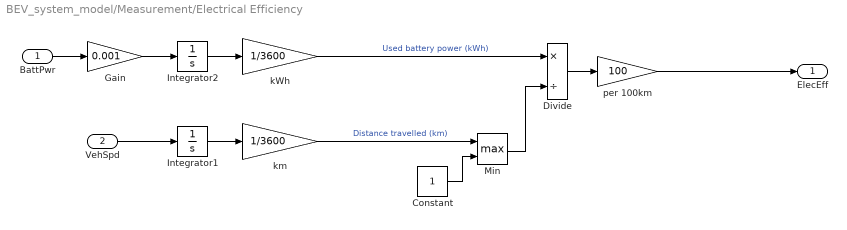
== system BEV_system_model/Measurement/Electrical Efficiency ==
  BattPwr : Inport  Unit=w
  VehSpd : Inport  Port=2  Unit=km/hr
  Constant : Constant
  Divide : Product  Inputs=*/
  Gain : Gain  Gain=0.001
  Integrator1 : Integrator
  Integrator2 : Integrator
  Min : MinMax  Function=max  Inputs=2
  kWh : Gain  Gain=1/3600
  km : Gain  Gain=1/3600
  per 100km : Gain  Gain=100
  ElecEff : Outport  Unit=kW*hr/(100*km)
  wires:
  km/1 -> Min/1  "Distance travelled (km)"
  Constant/1 -> Min/2
  Integrator2/1 -> kWh/1
  Divide/1 -> per 100km/1
  Integrator1/1 -> km/1
  Min/1 -> Divide/2
  kWh/1 -> Divide/1  "Used battery power (kWh)"
  per 100km/1 -> ElecEff/1
  VehSpd/1 -> Integrator1/1
  Gain/1 -> Integrator2/1
  BattPwr/1 -> Gain/1
